simulink model "Non_Holonomical_Cubli"  (R2025b)
settings: Solver=ode15s  StartTime=0  StopTime=13  MaxStep=1e-3  MinStep=1e-8  RelTol=1e-3
values from neighbouring files (symbols this model uses):
  m = 1.219    [physical_parameters.mat]    (also in tuning_parameter_corner.mat; tuning_parameter_edge.mat)
undefined symbols (not defined in the file or in its folder): X, Y, Z
libraries: sm_lib x79, nesl_utility x10, simulink x5, simulink_extras x2
(part 1 of 3)
settings Model: Creator=S Sanjay  LastModifiedBy=S Sanjay
settings SolverCC: InitialStep=1e-3  MaxConsecutiveMinStep=1e4
settings DataIOCC: FinalStateName=Edge_Balance  InitialState=Edge_Balance  SaveOperatingPoint=on
settings SFSimCC: SimTargetLang=C++  SimDLTargetLibrary=mkl-dnn
settings ExplorerConfigSet: InternalSimMechanicsExplorerSettings=|
  | <ExplorerConfiguration>
  | 
  |   <canonicalview>default</canonicalview>
  | 
  |   <TilePanel>
  |     <TileInfo>
  |       <Tiles Columns="1" Count="1" Height="608" Rows="1" Width="1340">
  |         <Row Weight="1"/>
  |         <Column Weight="1"/>
  |         <Tile Height="1" Width="1" X="0" Y="0"/>
  |       </Tiles>
  |     </TileInfo>
  |     <SceneInfo>
  |       <SceneViewer>
  |         <IsThisViewStd>
  |           <IsStandardView>off</IsStandardView>
  |           <StandardViewName>Front</StandardViewName>
  |         </IsThisViewStd>
  |         <BGColor>
  |           <R>1</R>
  |           <G>1</G>
  |           <B>1</B>
  |           <A>1</A>
  |         </BGColor>
  |         <Camera>
  |           <DoPerspective>off</DoPerspective>
  |           <Position>
  |             <X>-0.040054821891673767</X>
  |             <Y>-0.70442291530903711</Y>
  |             <Z>0.071525398260554526</Z>
  |           </Position>
  |           <Center>
  |             <X>-0.040054821891673767</X>
  |             <Y>0.074999999999999997</Y>
  |             <Z>0.071525398260554526</Z>
  |           </Center>
  |           <Up>
  |             <X>0</X>
  |             <Y>0</Y>
  |             <Z>1</Z>
  |           </Up>
  |           <XLim>0.15052058136869881</XLim>
  |           <YLim>0.15052058136869881</YLim>
  |           <ViewLimDist>0.01</ViewLimDist>
  |         </Camera>
  |       </SceneViewer>
  |     </SceneInfo>
  |   </TilePanel>
  | 
  |   <MechEditorPanel>
  |     <GfxPanelCameraMap/>
  |     <Cameras/>
  |     <VideoCreator>
  |       <IncludeTiles>All</IncludeTiles>
  |       <IncludeTime>on</IncludeTime>
  |       <IncludeWorldFrame>off</IncludeWorldFrame>
  |       <PlaybackSpeedRatio>1</PlaybackSpeedRatio>
  |       <FrameRate>30</FrameRate>
  |       <FrameSize>[1280, 720]</FrameSize>
  |       <VideoFormat>MPEG4</VideoFormat>
  |     </VideoCreator>
  |   </MechEditorPanel>
  | 
  |   <PlaybackSettings>
  |     <PlaybackSpeedFactor>1</PlaybackSpeedFactor>
  |   </PlaybackSettings>
  | 
  | </ExplorerConfiguration>

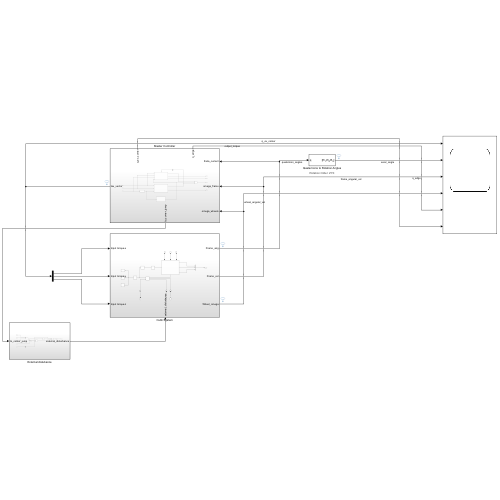
[thumbnail: Simulink's stored preview of the top-level diagram]
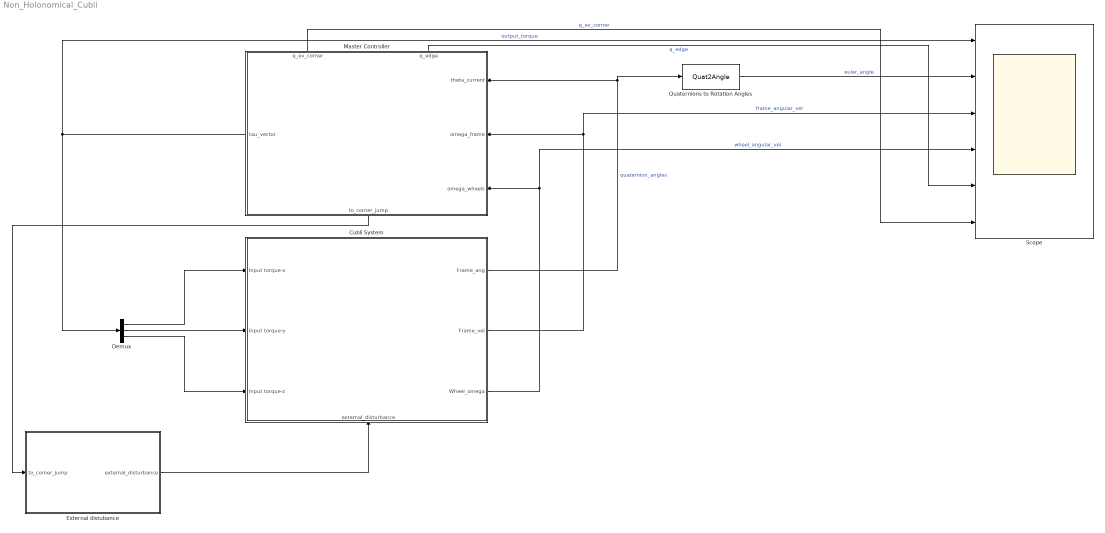
== system Non_Holonomical_Cubli ==
  Cubli System : Subsystem
      settings: PortSchema="{\"entries\":[{\"content\":{\"sides\":[{\"content\":{\"connectorIds\":[\"In1\",\"In2\",\"In3\"]},\"type\":\"ConnectorPlacement.EquallySpacedRectSide\",\"uuid\":\"5f5b9516-a4fd-4785-926f-66a98ec2aae9\"},{\"content\":{\"connectorIds\":[\"Out1\",\"Out2\",\"Out3\"],\"side\":\"RIGHT\"},\"type\":\"ConnectorPlacement.EquallySpacedRectSide\",\"uuid\":\"60d5ee22-f38f-41d5-b6d6-7b831adbf2a8\"},{\"content\":{\"side\":\"TOP\"},\"type\":\"ConnectorPlacement.EquallySpacedRectSide\",\"uuid\":\"7dec9ffc-12fc-4598-886c-49b3d3caf796\"},{\"content\":{\"connectorIds\":[\"In4\"],\"side\":\"BOTTOM\"},\"type\":\"ConnectorPlacement.EquallySpacedRectSide\",\"uuid\":\"6f94ea6b-f13b-4fc8-9dbe-3e3d3e7c7d3e\"}]},\"type\":\"ConnectorPlacement.EquallySpacedConnector\",\"uuid\":\"330043f2-5c26-4a0f-a502-bfb2b6aa9a82\"}],\"packageUris\":[\"http://schema.mathworks.com/mf0/Connector/R2020b\"],\"version\":\"1.0\"}"
  Demux : Demux  Outputs=3
  External distubance : Subsystem
  Master Controller : Subsystem
      settings: PortSchema="{\"entries\":[{\"content\":{\"sides\":[{\"content\":{\"connectorIds\":[\"In1\",\"In2\",\"In3\"]},\"type\":\"ConnectorPlacement.EquallySpacedRectSide\",\"uuid\":\"2cdceb7b-abfe-4398-b06f-eb5d2b1f6282\"},{\"content\":{\"connectorIds\":[\"Out1\"],\"side\":\"RIGHT\"},\"type\":\"ConnectorPlacement.EquallySpacedRectSide\",\"uuid\":\"01c339db-17ac-4119-86eb-536633adac2c\"},{\"content\":{\"connectorIds\":[\"Out3\",\"Out4\"],\"side\":\"TOP\"},\"type\":\"ConnectorPlacement.EquallySpacedRectSide\",\"uuid\":\"b96001bd-d179-4ff4-a950-c514b8b3d76b\"},{\"content\":{\"connectorIds\":[\"Out2\"],\"side\":\"BOTTOM\"},\"type\":\"ConnectorPlacement.EquallySpacedRectSide\",\"uuid\":\"361f408d-891c-47d0-b8eb-9646463b4a1f\"}]},\"type\":\"ConnectorPlacement.EquallySpacedConnector\",\"uuid\":\"bf28b1fe-494a-4ec5-b1bb-391f95a1c354\"}],\"packageUris\":[\"http://schema.mathworks.com/mf0/Connector/R2020b\"],\"version\":\"1.0\"}"
  Quaternions to Rotation Angles : Quat2Angle
      settings: AttributesFormatString=Rotation Order: %<rotationOrder>
  Scope : Scope  NumInputPorts=6
      settings: ActiveDisplayYMinimum=-12.75  ActiveDisplayYMaximum=24.75
  wires:
  Cubli System/1(Frame_ang) -> Quaternions to Rotation Angles/1, Master Controller/1(theta_current)  "quaternion_angles"
  Cubli System/2(Frame_vel) -> Scope/3, Master Controller/2(omega_frame)  "frame_angular_vel"
  Cubli System/3(Wheel_omega) -> Scope/4, Master Controller/3(omega_wheels)  "wheel_angular_vel"
  Master Controller/1(tau_vector) -> Scope/1, Demux/1  "output_torque"
  Demux/1 -> Cubli System/1(Input torque-x)
  Demux/2 -> Cubli System/2(Input torque-y)
  Demux/3 -> Cubli System/3(Input torque-z)
  Master Controller/3(q_edge) -> Scope/5  "q_edge"
  Master Controller/4(q_ev_corner) -> Scope/6  "q_ev_corner"
  Quaternions to Rotation Angles/1 -> Scope/2  "euler_angle"
  Master Controller/2(to_corner_jump) -> External distubance/1(to_corner_jump)
  External distubance/1(external_disturbance) -> Cubli System/4(external_disturbance)

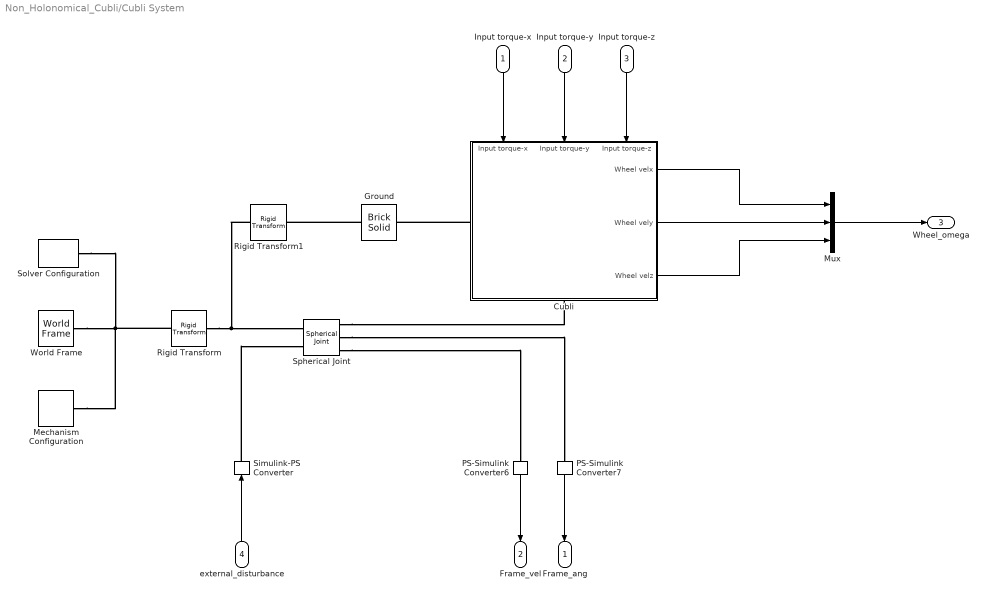
== system Non_Holonomical_Cubli/Cubli System ==
  Input torque-x : Inport
  Input torque-y : Inport  Port=2
  Input torque-z : Inport  Port=3
  external_disturbance : Inport  Port=4
  Cubli : Subsystem
      settings: PortSchema="{\"entries\":[{\"content\":{\"sides\":[{\"content\":{\"connectorIds\":[\"LConn1\"]},\"type\":\"ConnectorPlacement.EquallySpacedRectSide\",\"uuid\":\"6adf7ee2-c4b8-4796-ad09-ce5711974701\"},{\"content\":{\"connectorIds\":[\"Out1\",\"Out2\",\"Out3\"],\"side\":\"RIGHT\"},\"type\":\"ConnectorPlacement.EquallySpacedRectSide\",\"uuid\":\"91dc68f1-4c76-44e8-ad07-f96271bd7b17\"},{\"content\":{\"connectorIds\":[\"In1\",\"In2\",\"In3\"],\"side\":\"TOP\"},\"type\":\"ConnectorPlacement.EquallySpacedRectSide\",\"uuid\":\"30232ce5-1395-4c39-8bb0-085fb3773f51\"},{\"content\":{\"connectorIds\":[\"RConn1\"],\"side\":\"BOTTOM\"},\"type\":\"ConnectorPlacement.EquallySpacedRectSide\",\"uuid\":\"0f945396-4cf4-432c-84ba-6526ad05d30a\"}]},\"type\":\"ConnectorPlacement.EquallySpacedConnector\",\"uuid\":\"10f6f1ea-d2be-46df-87d0-79c43156557a\"}],\"packageUris\":[\"http://schema.mathworks.com/mf0/Connector/R2020b\"],\"version\":\"1.0\"}"
  Ground : sm_lib/Body Elements/Brick Solid  BrickDimensions=[1 1 0.02]  BrickDimensionsUnits=m  ExportEntireGeometry=on  InertiaType=CalculateFromGeometry  BasedOnType=Density  Density=1000  DensityUnits=kg/m^3  Mass=1  MassUnits=kg  CenterOfMass=[0 0 0]  CenterOfMassUnits=m  MomentsOfInertia=[1 1 1]  MomentsOfInertiaUnits=kg*m^2  ProductsOfInertia=[0 0 0]  ProductsOfInertiaUnits=kg*m^2  GraphicType=FromGeometry  MarkerShape=Sphere  MarkerSize=10  GraphicVisPropType=SimpleVisualProperties  GraphicDiffuseColor=[0.5 0.5 0.5]  GraphicOpacity=1  GraphicSpecularColor=[0.5 0.5 0.5 1.0]  GraphicAmbientColor=[0.15 0.15 0.15 1.0]  GraphicEmissiveColor=[0.0 0.0 0.0 1.0]  GraphicShininess=75  DoExposeReferenceFrame=on  SerializedFrames=<Frames/>
  Mechanism Configuration : sm_lib/Utilities/Mechanism Configuration  UniformGravity=Constant  GravityVector=[0 0 -9.80665]  GravityVectorUnits=m/s^2  LinearizationDelta=0.001  JointModeTransitionNonlinearIterations=2
  Mux : Mux  Inputs=3
  PS-Simulink Converter6 : nesl_utility/PS-Simulink Converter  PhysicalDomain=network_engine_domain  SubClassName=ps_output  LeftPortType=input  RightPortType=output  PseudoPeriodic=off  Frequencies=[]  VectorFormat=inherit  Unit=inherit  AffineConversion=off
  PS-Simulink Converter7 : nesl_utility/PS-Simulink Converter  PhysicalDomain=network_engine_domain  SubClassName=ps_output  LeftPortType=input  RightPortType=output  PseudoPeriodic=off  Frequencies=[]  VectorFormat=inherit  Unit=inherit  AffineConversion=off
  Rigid Transform : sm_lib/Frames and Transforms/Rigid Transform  RotationMethod=None  FollAlignAxisA=+X  BaseAlignAxisA=+Y  FollAlignAxisB=+Y  BaseAlignAxisB=+Z  RotationStandardAxis=+X  RotationAngle=90  RotationAngleUnits=deg  RotationArbitraryAxis=[0 0 1]  RotationSequenceAxes=FollowerAxes  RotationSequence=XYX  RotationSequenceAngles=[90 180 0]  RotationSequenceAnglesUnits=deg  RotationMatrix=[1 0 0;0 1 0;0 0 1]  Quaternion=[1 0 0 0]  TranslationMethod=None  TranslationCartesianOffset=[0 0 0]  TranslationCartesianOffsetUnits=m  TranslationStandardAxis=+Z  TranslationStandardOffset=0  TranslationStandardOffsetUnits=m  TranslationROffset=0  TranslationROffsetUnits=m  TranslationThetaOffset=0  TranslationThetaOffsetUnits=deg  TranslationZOffset=0  TranslationZOffsetUnits=m
  Rigid Transform1 : sm_lib/Frames and Transforms/Rigid Transform  RotationMethod=None  FollAlignAxisA=+X  BaseAlignAxisA=+Y  FollAlignAxisB=+Y  BaseAlignAxisB=+Z  RotationStandardAxis=+X  RotationAngle=90  RotationAngleUnits=deg  RotationArbitraryAxis=[0 0 1]  RotationSequenceAxes=FollowerAxes  RotationSequence=XYX  RotationSequenceAngles=[90 180 0]  RotationSequenceAnglesUnits=deg  RotationMatrix=[1 0 0;0 1 0;0 0 1]  Quaternion=[1 0 0 0]  TranslationMethod=StandardAxis  TranslationCartesianOffset=[0 0 0]  TranslationCartesianOffsetUnits=m  TranslationStandardAxis=+Z  TranslationStandardOffset=-0.01  TranslationStandardOffsetUnits=m  TranslationROffset=0  TranslationROffsetUnits=m  TranslationThetaOffset=0  TranslationThetaOffsetUnits=deg  TranslationZOffset=0  TranslationZOffsetUnits=m
  Simulink-PS Converter : nesl_utility/Simulink-PS Converter  PhysicalDomain=network_engine_domain  SubClassName=ps_input  LeftPortType=input  RightPortType=output  PseudoPeriodic=off  Frequencies=[]  NoiseDistribution=none  NoiseParameters=[]  Unit=1  AffineConversion=off  FilteringAndDerivatives=provide  SimscapeFilterOrder=1  InputFilterTimeConstant=0.001  UdotUserProvided=0
  Solver Configuration : nesl_utility/Solver Configuration  PhysicalDomain=network_engine_domain  SubClassName=solver  LeftPortType=input  RightPortType=generic  Tones=[]  Harmonics=[]  SimulateNoise=off  Profile=off  UseLocalSampling=off  EnableSwitchedLinearOptims=on  FrequencyDomain=off  UseCCode=off  RelTol=0.001  AbsTol=0.001  MinStep=1e-09  ToWorkspace=off  RevertToSquareIcSolve=off  NumHomotopyIterations=100  PhasorMode=off  PhasorModeNumHarmonics=1  ConsistencySolver=NEWTON_XTOL_AFTER_FTOL  IndexReductionMethod=DerivativeReplacement  DoDC=off  ResidualTolerance=1e-09  ConsistencyTolSource=GLOBAL  ConsistencyAbsTol=0.001  ConsistencyRelTol=0.001  ConsistencyTolFactor=0.001  UseLocalSolver=off  LocalSolverChoice=NE_BACKWARD_EULER_ADVANCER  ResolveIndetEquations=on  FunctionEvalNumThread=1  LocalSolverSampleTime=0.001  DoFixedCost=off  MaxNonlinIter=3  MaxModeIter=2  ComputeImpulses=off  ImpulseIterations=2  LinearAlgebra=auto  LinearAlgebraNumThread=0  EquationFormulation=NE_TIME_EF  DelaysMemoryBudget=1024  AutomaticFiltering=on  FilteringTimeConstant=0.001  PartitionStorageMethod=AS_NEEDED  PartitionMemoryBudget=1024  PartitionMethod=ROBUST  MultibodyUseLocalSolver=off  MultibodyLocalSolverChoice=ODE1  MultibodyLocalSolverSampleTime=0.001
  Spherical Joint : sm_lib/Joints/Spherical Joint  JointMode=Normal  CompositeWrenchDir=FollowerOnBase  CompositeWrenchFrame=BaseFrame  SenseConstraintForce=off  SenseConstraintTorque=off  SenseTotalForce=off  SenseTotalTorque=off  PositionTargetSpecify=on  PositionTargetPriority=High  PositionTargetRotationMethod=RotationSequence  PositionTargetFollAlignAxisA=+X  PositionTargetBaseAlignAxisA=+Y  PositionTargetFollAlignAxisB=+Y  PositionTargetBaseAlignAxisB=+Z  PositionTargetRotationStandardAxis=+Z  PositionTargetRotationAngle=0  PositionTargetRotationAngleUnits=deg  PositionTargetRotationArbitraryAxis=[0 0 1]  PositionTargetRotationSequenceAxes=BaseAxes  PositionTargetRotationSequence=XYX  PositionTargetRotationSequenceAngles=[0 -05 0]  PositionTargetRotationSequenceAnglesUnits=deg  PositionTargetRotationMatrix=[1 0 0;0 1 0;0 0 1]  PositionTargetQuaternion=[1 0 0 0]  VelocityTargetSpecify=off  VelocityTargetPriority=High  VelocityTargetValue=[7.592 0.1228 0.0118]  VelocityTargetValueUnits=rad/s  VelocityTargetInFollowerFrame=off  EqPosRotationMethod=None  EqPosFollAlignAxisA=+X  EqPosBaseAlignAxisA=+Y  EqPosFollAlignAxisB=+Y  EqPosBaseAlignAxisB=+Z  EqPosRotationStandardAxis=+Z  EqPosRotationAngle=0  EqPosRotationAngleUnits=deg  EqPosRotationArbitraryAxis=[0 0 1]  EqPosRotationSequenceAxes=FollowerAxes  EqPosRotationSequence=XYX  EqPosRotationSequenceAngles=[0 0 0]  EqPosRotationSequenceAnglesUnits=deg  EqPosRotationMatrix=[1 0 0;0 1 0;0 0 1]  EqPosQuaternion=[1 0 0 0]  SpringStiffness=0  SpringStiffnessUnits=N*m/deg  DampingCoefficient=0.01  DampingCoefficientUnits=N*m/(deg/s)  LowerLimitSpecify=off  LowerLimitBound=15  LowerLimitBoundUnits=deg  LowerLimitStiffness=1e4  LowerLimitStiffnessUnits=N*m/deg  LowerLimitDamping=10  LowerLimitDampingUnits=N*m/(deg/s)  LowerLimitTransitionRegionWidth=0.1  LowerLimitTransitionRegionWidthUnits=deg  UpperLimitSpecify=off  UpperLimitBound=45  UpperLimitBoundUnits=deg  UpperLimitStiffness=1e4  UpperLimitStiffnessUnits=N*m/deg  UpperLimitDamping=10  UpperLimitDampingUnits=N*m/(deg/s)  UpperLimitTransitionRegionWidth=0.1  UpperLimitTransitionRegionWidthUnits=deg  TorqueActuationMode=InputTorque  ActuateTorqueX=off  ActuateTorqueY=off  ActuateTorqueZ=off  ActuateTorque=on  ActuationFrame=BaseFrame  SensePosition=on  SenseVelocityX=off  SenseVelocityY=off  SenseVelocityZ=off  SenseVelocity=on  SenseAccelerationX=off  SenseAccelerationY=off  SenseAccelerationZ=off  SenseAcceleration=off  SenseLowerLimitTorqueMag=off  SenseUpperLimitTorqueMag=off  SensingFrame=BaseFrame
  World Frame : sm_lib/Frames and Transforms/World Frame
  Frame_ang : Outport
  Frame_vel : Outport  Port=2
  Wheel_omega : Outport  Port=3
  wires:
  Input torque-z/1 -> Cubli/3(Input torque-z)
  Input torque-y/1 -> Cubli/2(Input torque-y)
  Input torque-x/1 -> Cubli/1(Input torque-x)
  Cubli/2(Wheel vely) -> Mux/2
  Cubli/1(Wheel velx) -> Mux/1
  Cubli/3(Wheel velz) -> Mux/3
  Mux/1 -> Wheel_omega/1
  PS-Simulink Converter6/1 -> Frame_vel/1
  PS-Simulink Converter7/1 -> Frame_ang/1
  external_disturbance/1 -> Simulink-PS Converter/1
  connections:
  World Frame/RConn1 -- Rigid Transform/LConn1 -- Solver Configuration/RConn1 -- Mechanism Configuration/RConn1
  Spherical Joint/RConn1 -- Cubli/RConn1
  Rigid Transform/RConn1 -- Rigid Transform1/LConn1 -- Spherical Joint/LConn1
  Spherical Joint/RConn3 -- PS-Simulink Converter6/LConn1
  Spherical Joint/RConn2 -- PS-Simulink Converter7/LConn1
  Ground/RConn1 -- Rigid Transform1/RConn1
  Cubli/LConn1 -- Ground/LConn1
  Simulink-PS Converter/RConn1 -- Spherical Joint/LConn2

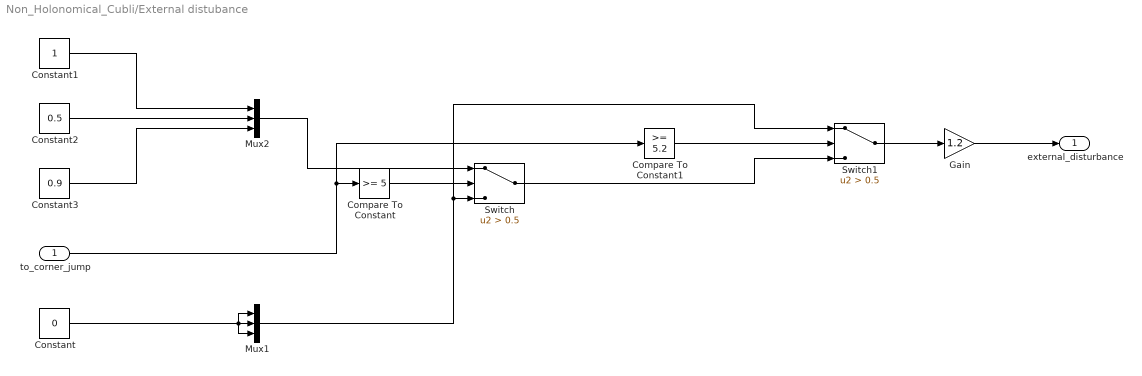
== system Non_Holonomical_Cubli/External distubance ==
  to_corner_jump : Inport
  Compare To Constant : simulink/Logic and Bit Operations/Compare To Constant  relop=>=  const=5  OutDataTypeStr=boolean
  Compare To Constant1 : simulink/Logic and Bit Operations/Compare To Constant  relop=>=  const=5.2  OutDataTypeStr=boolean
  Constant : Constant  Value=0
  Constant1 : Constant
  Constant2 : Constant  Value=0.5
  Constant3 : Constant  Value=0.9
  Gain : Gain  Gain=1.2
  Mux1 : Mux  Inputs=3
  Mux2 : Mux  Inputs=3
  Switch : Switch  Criteria=u2 > Threshold  Threshold=0.5  SaturateOnIntegerOverflow=off  InputSameDT=off
  Switch1 : Switch  Criteria=u2 > Threshold  Threshold=0.5  SaturateOnIntegerOverflow=off  InputSameDT=off
  external_disturbance : Outport
  wires:
  Compare To Constant/1 -> Switch/2
  to_corner_jump/1 -> Compare To Constant/1, Compare To Constant1/1
  Switch/1 -> Switch1/3
  Constant1/1 -> Mux2/1
  Constant/1 -> Mux1/3, Mux1/1, Mux1/2
  Mux1/1 -> Switch1/1, Switch/3
  Compare To Constant1/1 -> Switch1/2
  Constant2/1 -> Mux2/2
  Constant3/1 -> Mux2/3
  Switch1/1 -> Gain/1
  Mux2/1 -> Switch/1
  Gain/1 -> external_disturbance/1

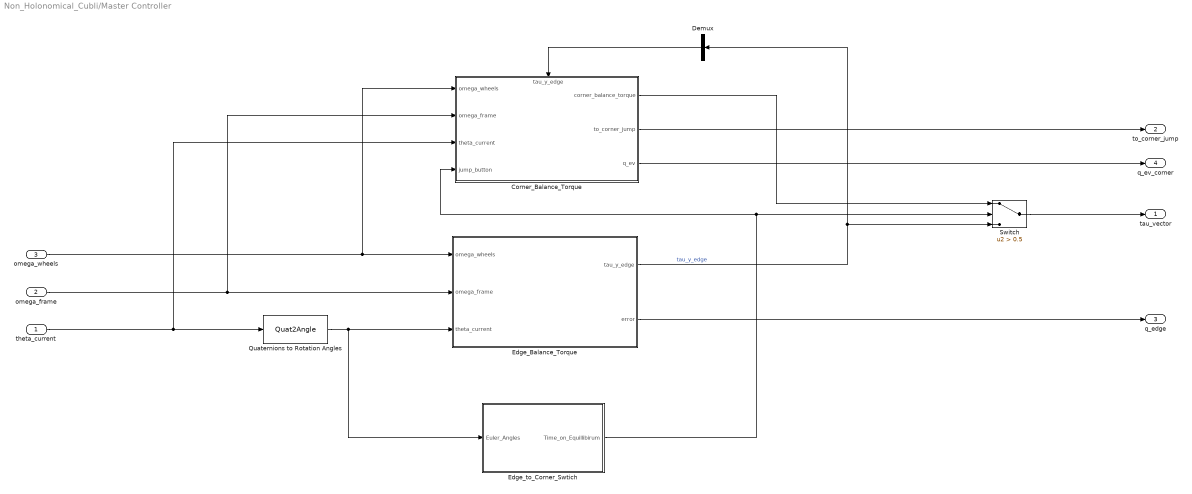
== system Non_Holonomical_Cubli/Master Controller ==
  theta_current : Inport
  omega_frame : Inport  Port=2
  omega_wheels : Inport  Port=3
  Corner_Balance_Torque : Subsystem
      settings: PortSchema="{\"entries\":[{\"content\":{\"sides\":[{\"content\":{\"connectorIds\":[\"In1\",\"In2\",\"In3\",\"In4\"]},\"type\":\"ConnectorPlacement.EquallySpacedRectSide\",\"uuid\":\"1f7b0852-8b9a-4eba-b230-002f04ce1124\"},{\"content\":{\"connectorIds\":[\"Out1\",\"Out2\",\"Out3\"],\"side\":\"RIGHT\"},\"type\":\"ConnectorPlacement.EquallySpacedRectSide\",\"uuid\":\"21919282-dafc-4587-878f-e5107e503542\"},{\"content\":{\"connectorIds\":[\"In5\"],\"side\":\"TOP\"},\"type\":\"ConnectorPlacement.EquallySpacedRectSide\",\"uuid\":\"4f05e2a3-4b7f-447f-b0fe-b8f447574882\"}]},\"type\":\"ConnectorPlacement.EquallySpacedConnector\",\"uuid\":\"49aab782-7a49-4f61-ae94-efa1138c681a\"}],\"packageUris\":[\"http://schema.mathworks.com/mf0/Connector/R2020b\"],\"version\":\"1.0\"}"
  Demux : Demux  Outputs=3
  Edge_Balance_Torque : Subsystem
  Edge_to_Corner_Swtich : Subsystem
  Quaternions to Rotation Angles : Quat2Angle
      settings: AttributesFormatString=Rotation Order: %<rotationOrder>
  Switch : Switch  Criteria=u2 > Threshold  Threshold=0.5  SaturateOnIntegerOverflow=off  InputSameDT=off
  tau_vector : Outport
  to_corner_jump : Outport  Port=2
  q_edge : Outport  Port=3
  q_ev_corner : Outport  Port=4
  wires:
  omega_frame/1 -> Corner_Balance_Torque/2(omega_frame), Edge_Balance_Torque/2(omega_frame)
  omega_wheels/1 -> Corner_Balance_Torque/1(omega_wheels), Edge_Balance_Torque/1(omega_wheels)
  Edge_Balance_Torque/2(error) -> q_edge/1
  theta_current/1 -> Quaternions to Rotation Angles/1, Corner_Balance_Torque/3(theta_current)
  Quaternions to Rotation Angles/1 -> Edge_to_Corner_Swtich/1(Euler_Angles), Edge_Balance_Torque/3(theta_current)
  Corner_Balance_Torque/1(corner_balance_torque) -> Switch/1
  Switch/1 -> tau_vector/1
  Edge_to_Corner_Swtich/1(Time_on_Equillibirum) -> Switch/2, Corner_Balance_Torque/4(jump_button)
  Edge_Balance_Torque/1(tau_y_edge) -> Demux/1, Switch/3  "tau_y_edge"
  Demux/2 -> Corner_Balance_Torque/5(tau_y_edge)
  Corner_Balance_Torque/2(to_corner_jump) -> to_corner_jump/1
  Corner_Balance_Torque/3(q_ev) -> q_ev_corner/1

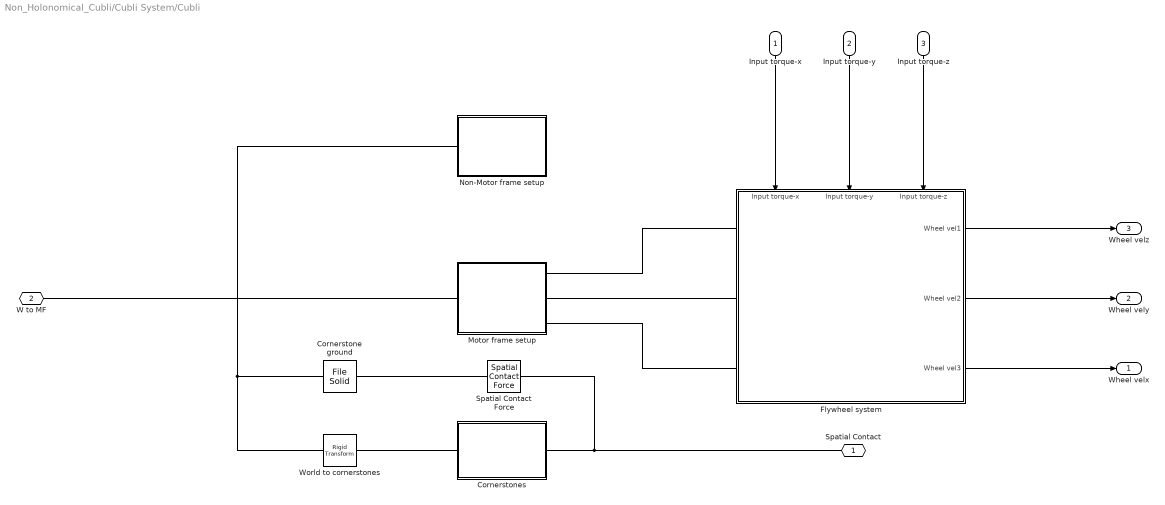
== system Non_Holonomical_Cubli/Cubli System/Cubli ==
  Input torque-x : Inport
  Input torque-y : Inport  Port=2
  Input torque-z : Inport  Port=3
  Cornerstone ground : sm_lib/Body Elements/File Solid  ExtGeomFileName=D:\Mechatronics\Non-Holonomical Cubli\GitHub Referance\balancing-cube-main\mechanical\models\cornerstone-b.step  UnitType=FromFile  ExtGeomFileUnits=m  StepReaderType=HEX  ExportConvexHullGeometry=on  InertiaType=Custom  BasedOnType=DensityFromFile  Density=1000  DensityUnits=kg/m^3  Mass=15.195  MassUnits=g  CenterOfMass=[7.102 7.102 7.102]  CenterOfMassUnits=mm  MomentsOfInertia=[4.91955e-7 4.91955e-7 4.91955e-7]  MomentsOfInertiaUnits=kg*m^2  ProductsOfInertia=[2.9611e-8 2.9611e-8 2.9611e-8]  ProductsOfInertiaUnits=kg*m^2  GraphicType=FromGeometry  MarkerShape=Sphere  MarkerSize=10  GraphicVisPropType=SimpleVisualProperties  GraphicDiffuseColor=[0 0.7137 0.02353]  GraphicOpacity=1  GraphicSpecularColor=[0.5 0.5 0.5 1.0]  GraphicAmbientColor=[0.15 0.15 0.15 1.0]  GraphicEmissiveColor=[0.0 0.0 0.0 1.0]  GraphicShininess=75  DoExposeReferenceFrame=on  SerializedFrames=<Frames/>
  Cornerstones : Subsystem
  Flywheel system : Subsystem
      settings: PortSchema="{\"entries\":[{\"content\":{\"sides\":[{\"content\":{\"connectorIds\":[\"LConn1\",\"LConn2\",\"LConn3\"]},\"type\":\"ConnectorPlacement.EquallySpacedRectSide\",\"uuid\":\"bd01766a-4f70-4c8a-b3da-7a2c61393a0a\"},{\"content\":{\"connectorIds\":[\"Out1\",\"Out2\",\"Out3\"],\"side\":\"RIGHT\"},\"type\":\"ConnectorPlacement.EquallySpacedRectSide\",\"uuid\":\"6c934dc6-4dcb-4252-8a96-3382836f91aa\"},{\"content\":{\"connectorIds\":[\"In1\",\"In2\",\"In3\"],\"side\":\"TOP\"},\"type\":\"ConnectorPlacement.EquallySpacedRectSide\",\"uuid\":\"3baafda2-b803-466a-93fa-ff8a48a98b9a\"}]},\"type\":\"ConnectorPlacement.EquallySpacedConnector\",\"uuid\":\"eb6514d5-6f26-4cfd-b495-999f94607100\"}],\"packageUris\":[\"http://schema.mathworks.com/mf0/Connector/R2020b\"],\"version\":\"1.0\"}"
  Motor frame setup : Subsystem
  Non-Motor frame setup : Subsystem
  Spatial Contact Force : sm_lib/Forces and Torques/Spatial Contact Force  SenseSeparationDistance=off  NormalForceType=SmoothSpringDamper  NormalStiffness=1e6  NormalStiffnessUnits=N/m  NormalDamping=1e3  NormalDampingUnits=N/(m/s)  NormalTransitionRegionWidth=1e-4  NormalTransitionRegionWidthUnits=m  FrictionType=SmoothStickSlip  CoefficientOfStaticFriction=0.5  CoefficientOfDynamicFriction=0.3  FrictionalCriticalVelocity=1e-3  FrictionalCriticalVelocityUnits=m/s  SenseContactSignal=off  SensePenetrationDepth=off  SenseNormalVelocity=off  SenseTangentialVelocity=off  SensingForceTorqueDirection=BaseOnFollower  SensingForceTorqueResolutionFrame=ContactFrame  SenseNormalForce=off  SenseNormalForceMagnitude=off  SenseNormalTorque=off  SenseFrictionalForce=off  SenseFrictionalForceMagnitude=off  SenseFrictionalTorque=off  SenseTotalForce=off  SenseTotalTorque=off  SenseContactBaseRotation=off  SenseContactBaseTranslation=off  SenseContactFollowerRotation=off  SenseContactFollowerTranslation=off  ZeroCrossDetectContactStartAndEnd=off
  World to cornerstones : sm_lib/Frames and Transforms/Rigid Transform  RotationMethod=StandardAxis  FollAlignAxisA=+X  BaseAlignAxisA=+Y  FollAlignAxisB=+Y  BaseAlignAxisB=+Z  RotationStandardAxis=+Z  RotationAngle=180  RotationAngleUnits=deg  RotationArbitraryAxis=[0 0 1]  RotationSequenceAxes=FollowerAxes  RotationSequence=XZY  RotationSequenceAngles=[0 0 0]  RotationSequenceAnglesUnits=deg  RotationMatrix=[1 0 0;0 1 0;0 0 1]  Quaternion=[1 0 0 0]  TranslationMethod=Cartesian  TranslationCartesianOffset=[75 75 0]  TranslationCartesianOffsetUnits=mm  TranslationStandardAxis=+Z  TranslationStandardOffset=0  TranslationStandardOffsetUnits=m  TranslationROffset=0  TranslationROffsetUnits=m  TranslationThetaOffset=0  TranslationThetaOffsetUnits=deg  TranslationZOffset=0  TranslationZOffsetUnits=m
  Spatial Contact : PMIOPort  Side=Left
  W to MF : PMIOPort  Port=2  Side=Right
  Wheel velx : Outport
  Wheel vely : Outport  Port=2
  Wheel velz : Outport  Port=3
  wires:
  Flywheel system/1(Wheel vel1) -> Wheel velz/1
  Input torque-z/1 -> Flywheel system/3(Input torque-z)
  Flywheel system/3(Wheel vel3) -> Wheel velx/1
  Flywheel system/2(Wheel vel2) -> Wheel vely/1
  Input torque-x/1 -> Flywheel system/1(Input torque-x)
  Input torque-y/1 -> Flywheel system/2(Input torque-y)
  connections:
  World to cornerstones/LConn1 -- Non-Motor frame setup/LConn1 -- W to MF/RConn1 -- Motor frame setup/LConn1 -- Cornerstone ground/RConn1
  Cornerstones/LConn1 -- World to cornerstones/RConn1
  Flywheel system/LConn2 -- Motor frame setup/RConn2
  Flywheel system/LConn1 -- Motor frame setup/RConn1
  Flywheel system/LConn3 -- Motor frame setup/RConn3
  Spatial Contact/RConn1 -- Spatial Contact Force/LConn1 -- Cornerstones/RConn1
  Spatial Contact Force/RConn1 -- Cornerstone ground/LConn1

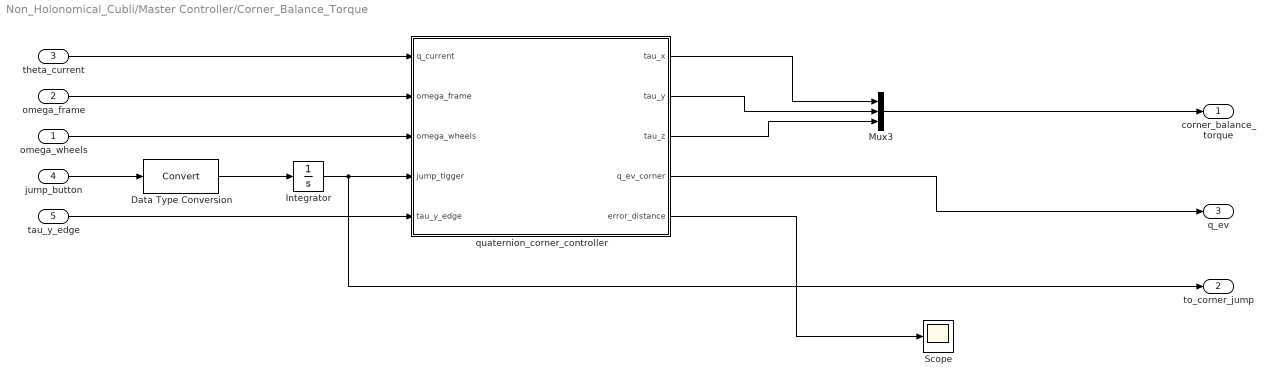
== system Non_Holonomical_Cubli/Master Controller/Corner_Balance_Torque ==
  omega_wheels : Inport
  omega_frame : Inport  Port=2
  theta_current : Inport  Port=3
  jump_button : Inport  Port=4
  tau_y_edge : Inport  Port=5
  Data Type Conversion : DataTypeConversion  SaturateOnIntegerOverflow=off  RndMeth=Floor
  Integrator : Integrator
  Mux3 : Mux  Inputs=3
  Scope : Scope
      settings: ActiveDisplayYMinimum=-0.059292060386496544  ActiveDisplayYMaximum=0.53363013219783351
  quaternion_corner_controller : MATLAB Function  TreatAsAtomicUnit=on
  corner_balance_torque : Outport
  to_corner_jump : Outport  Port=2
  q_ev : Outport  Port=3
  wires:
  omega_frame/1 -> quaternion_corner_controller/2(omega_frame)
  omega_wheels/1 -> quaternion_corner_controller/3(omega_wheels)
  quaternion_corner_controller/2(tau_y) -> Mux3/2
  quaternion_corner_controller/1(tau_x) -> Mux3/1
  quaternion_corner_controller/3(tau_z) -> Mux3/3
  Mux3/1 -> corner_balance_torque/1
  tau_y_edge/1 -> quaternion_corner_controller/5(tau_y_edge)
  jump_button/1 -> Data Type Conversion/1
  Integrator/1 -> to_corner_jump/1, quaternion_corner_controller/4(jump_tigger)
  Data Type Conversion/1 -> Integrator/1
  theta_current/1 -> quaternion_corner_controller/1(q_current)
  quaternion_corner_controller/4(q_ev_corner) -> q_ev/1
  quaternion_corner_controller/5(error_distance) -> Scope/1

== system Non_Holonomical_Cubli/Master Controller/Edge_Balance_Torque ==
  omega_wheels : Inport
  omega_frame : Inport  Port=2
  theta_current : Inport  Port=3
  Edge_SMC : MATLAB Function  TreatAsAtomicUnit=on
  Mux : Mux  Inputs=3
  jump_switch : Subsystem
  tau_y_edge : Outport
  error : Outport  Port=2
  wires:
  Edge_SMC/4(error_distance) -> error/1
  omega_frame/1 -> Edge_SMC/2(omega_frame)
  omega_wheels/1 -> Edge_SMC/3(omega_wheels)
  theta_current/1 -> jump_switch/1(theta_angle), Edge_SMC/1(theta_current)
  Edge_SMC/2(tau_y) -> Mux/2
  Edge_SMC/1(tau_x) -> Mux/1
  Edge_SMC/3(tau_z) -> Mux/3
  jump_switch/1(timmer) -> Edge_SMC/4(jump_trigger)
  Mux/1 -> tau_y_edge/1

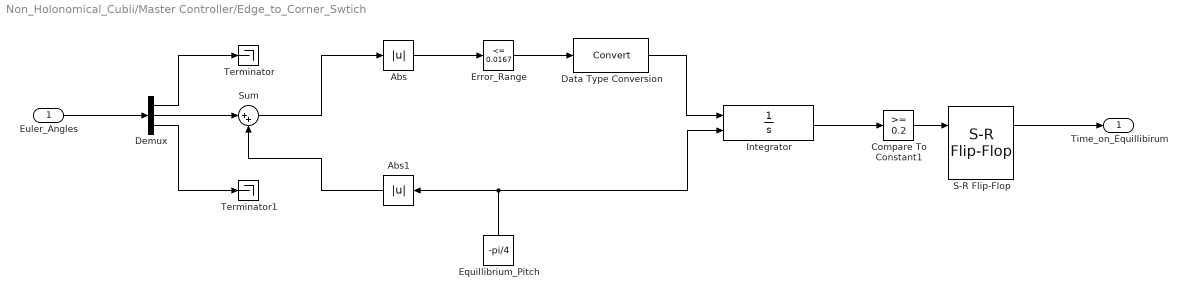
== system Non_Holonomical_Cubli/Master Controller/Edge_to_Corner_Swtich ==
  Euler_Angles : Inport
  Abs : Abs  SaturateOnIntegerOverflow=off
  Abs1 : Abs  SaturateOnIntegerOverflow=off
  Compare To Constant1 : simulink/Logic and Bit Operations/Compare To Constant  relop=>=  const=0.2  OutDataTypeStr=boolean
  Data Type Conversion : DataTypeConversion  SaturateOnIntegerOverflow=off  RndMeth=Floor
  Demux : Demux  Outputs=3
  Equillibrium_Pitch : Constant  Value=-pi/4
  Error_Range : simulink/Logic and Bit Operations/Compare To Constant  relop=<=  const=0.0167  OutDataTypeStr=boolean
  Integrator : Integrator  ExternalReset=falling
  S-R Flip-Flop : simulink_extras/Flip Flops/S-R Flip-Flop  initial_condition=0
  Sum : Sum  Inputs=|++
  Terminator : Terminator
  Terminator1 : Terminator
  Time_on_Equillibirum : Outport
  wires:
  Compare To Constant1/1 -> S-R Flip-Flop/1
  Equillibrium_Pitch/1 -> Integrator/2, Abs1/1
  Abs/1 -> Error_Range/1
  Abs1/1 -> Sum/2
  Data Type Conversion/1 -> Integrator/1
  Error_Range/1 -> Data Type Conversion/1
  Demux/2 -> Sum/1
  Integrator/1 -> Compare To Constant1/1
  Sum/1 -> Abs/1
  Demux/3 -> Terminator1/1
  Demux/1 -> Terminator/1
  S-R Flip-Flop/1 -> Time_on_Equillibirum/1
  Euler_Angles/1 -> Demux/1

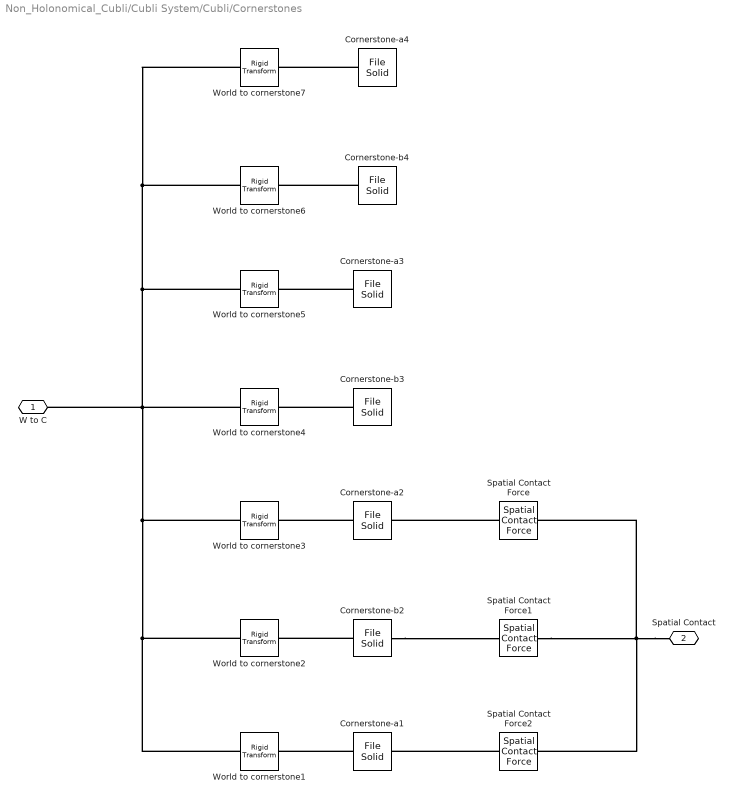
== system Non_Holonomical_Cubli/Cubli System/Cubli/Cornerstones ==
  Cornerstone-a1 : sm_lib/Body Elements/File Solid  ExtGeomFileName=D:\Mechatronics\Non-Holonomical Cubli\GitHub Referance\balancing-cube-main\mechanical\models\cornerstone-a.step  UnitType=FromFile  ExtGeomFileUnits=m  StepReaderType=HEX  ExportConvexHullGeometry=on  InertiaType=Custom  BasedOnType=DensityFromFile  Density=1000  DensityUnits=kg/m^3  Mass=15.195  MassUnits=g  CenterOfMass=[7.102 7.102 7.102]  CenterOfMassUnits=mm  MomentsOfInertia=[4.91955e-7 4.91955e-7 4.91955e-7]  MomentsOfInertiaUnits=kg*m^2  ProductsOfInertia=[2.9611e-8 2.9611e-8 2.9611e-8]  ProductsOfInertiaUnits=kg*m^2  GraphicType=FromGeometry  MarkerShape=Sphere  MarkerSize=10  GraphicVisPropType=SimpleVisualProperties  GraphicDiffuseColor=[0 0.7137 0.02353]  GraphicOpacity=1  GraphicSpecularColor=[0.5 0.5 0.5 1.0]  GraphicAmbientColor=[0.15 0.15 0.15 1.0]  GraphicEmissiveColor=[0.0 0.0 0.0 1.0]  GraphicShininess=75  DoExposeReferenceFrame=on  SerializedFrames=<Frames/>
  Cornerstone-a2 : sm_lib/Body Elements/File Solid  ExtGeomFileName=D:\Mechatronics\Non-Holonomical Cubli\GitHub Referance\balancing-cube-main\mechanical\models\cornerstone-a.step  UnitType=FromFile  ExtGeomFileUnits=m  StepReaderType=HEX  ExportConvexHullGeometry=on  InertiaType=Custom  BasedOnType=DensityFromFile  Density=1000  DensityUnits=kg/m^3  Mass=15.195  MassUnits=g  CenterOfMass=[7.102 7.102 7.102]  CenterOfMassUnits=mm  MomentsOfInertia=[4.91955e-7 4.91955e-7 4.91955e-7]  MomentsOfInertiaUnits=kg*m^2  ProductsOfInertia=[2.9611e-8 2.9611e-8 2.9611e-8]  ProductsOfInertiaUnits=kg*m^2  GraphicType=FromGeometry  MarkerShape=Sphere  MarkerSize=10  GraphicVisPropType=SimpleVisualProperties  GraphicDiffuseColor=[0 0.7137 0.02353]  GraphicOpacity=1  GraphicSpecularColor=[0.5 0.5 0.5 1.0]  GraphicAmbientColor=[0.15 0.15 0.15 1.0]  GraphicEmissiveColor=[0.0 0.0 0.0 1.0]  GraphicShininess=75  DoExposeReferenceFrame=on  SerializedFrames=<Frames/>
  Cornerstone-a3 : sm_lib/Body Elements/File Solid  ExtGeomFileName=D:\Mechatronics\Non-Holonomical Cubli\GitHub Referance\balancing-cube-main\mechanical\models\cornerstone-a.step  UnitType=FromFile  ExtGeomFileUnits=m  StepReaderType=HEX  ExportConvexHullGeometry=off  InertiaType=Custom  BasedOnType=DensityFromFile  Density=1000  DensityUnits=kg/m^3  Mass=15.195  MassUnits=g  CenterOfMass=[7.102 7.102 7.102]  CenterOfMassUnits=mm  MomentsOfInertia=[4.91955e-7 4.91955e-7 4.91955e-7]  MomentsOfInertiaUnits=kg*m^2  ProductsOfInertia=[2.9611e-8 2.9611e-8 2.9611e-8]  ProductsOfInertiaUnits=kg*m^2  GraphicType=FromGeometry  MarkerShape=Sphere  MarkerSize=10  GraphicVisPropType=SimpleVisualProperties  GraphicDiffuseColor=[0 0.7137 0.02353]  GraphicOpacity=1  GraphicSpecularColor=[0.5 0.5 0.5 1.0]  GraphicAmbientColor=[0.15 0.15 0.15 1.0]  GraphicEmissiveColor=[0.0 0.0 0.0 1.0]  GraphicShininess=75  DoExposeReferenceFrame=on  SerializedFrames=<Frames/>
  Cornerstone-a4 : sm_lib/Body Elements/File Solid  ExtGeomFileName=D:\Mechatronics\Non-Holonomical Cubli\GitHub Referance\balancing-cube-main\mechanical\models\cornerstone-a.step  UnitType=FromFile  ExtGeomFileUnits=m  StepReaderType=HEX  ExportConvexHullGeometry=off  InertiaType=Custom  BasedOnType=DensityFromFile  Density=1000  DensityUnits=kg/m^3  Mass=15.195  MassUnits=g  CenterOfMass=[7.102 7.102 7.102]  CenterOfMassUnits=mm  MomentsOfInertia=[4.91955e-7 4.91955e-7 4.91955e-7]  MomentsOfInertiaUnits=kg*m^2  ProductsOfInertia=[2.9611e-8 2.9611e-8 2.9611e-8]  ProductsOfInertiaUnits=kg*m^2  GraphicType=FromGeometry  MarkerShape=Sphere  MarkerSize=10  GraphicVisPropType=SimpleVisualProperties  GraphicDiffuseColor=[0 0.7137 0.02353]  GraphicOpacity=1  GraphicSpecularColor=[0.5 0.5 0.5 1.0]  GraphicAmbientColor=[0.15 0.15 0.15 1.0]  GraphicEmissiveColor=[0.0 0.0 0.0 1.0]  GraphicShininess=75  DoExposeReferenceFrame=on  SerializedFrames=<Frames/>
  Cornerstone-b2 : sm_lib/Body Elements/File Solid  ExtGeomFileName=D:\Mechatronics\Non-Holonomical Cubli\GitHub Referance\balancing-cube-main\mechanical\models\cornerstone-b.step  UnitType=FromFile  ExtGeomFileUnits=m  StepReaderType=HEX  ExportConvexHullGeometry=on  InertiaType=Custom  BasedOnType=DensityFromFile  Density=1000  DensityUnits=kg/m^3  Mass=15.195  MassUnits=g  CenterOfMass=[7.102 7.102 7.102]  CenterOfMassUnits=mm  MomentsOfInertia=[4.91955e-7 4.91955e-7 4.91955e-7]  MomentsOfInertiaUnits=kg*m^2  ProductsOfInertia=[2.9611e-8 2.9611e-8 2.9611e-8]  ProductsOfInertiaUnits=kg*m^2  GraphicType=FromGeometry  MarkerShape=Sphere  MarkerSize=10  GraphicVisPropType=SimpleVisualProperties  GraphicDiffuseColor=[0 0.7137 0.02353]  GraphicOpacity=1  GraphicSpecularColor=[0.5 0.5 0.5 1.0]  GraphicAmbientColor=[0.15 0.15 0.15 1.0]  GraphicEmissiveColor=[0.0 0.0 0.0 1.0]  GraphicShininess=75  DoExposeReferenceFrame=on  SerializedFrames=<Frames/>
  Cornerstone-b3 : sm_lib/Body Elements/File Solid  ExtGeomFileName=D:\Mechatronics\Non-Holonomical Cubli\GitHub Referance\balancing-cube-main\mechanical\models\cornerstone-b.step  UnitType=FromFile  ExtGeomFileUnits=m  StepReaderType=HEX  ExportConvexHullGeometry=off  InertiaType=Custom  BasedOnType=DensityFromFile  Density=1000  DensityUnits=kg/m^3  Mass=15.195  MassUnits=g  CenterOfMass=[7.102 7.102 7.102]  CenterOfMassUnits=mm  MomentsOfInertia=[4.91955e-7 4.91955e-7 4.91955e-7]  MomentsOfInertiaUnits=kg*m^2  ProductsOfInertia=[2.9611e-8 2.9611e-8 2.9611e-8]  ProductsOfInertiaUnits=kg*m^2  GraphicType=FromGeometry  MarkerShape=Sphere  MarkerSize=10  GraphicVisPropType=SimpleVisualProperties  GraphicDiffuseColor=[0 0.7137 0.02353]  GraphicOpacity=1  GraphicSpecularColor=[0.5 0.5 0.5 1.0]  GraphicAmbientColor=[0.15 0.15 0.15 1.0]  GraphicEmissiveColor=[0.0 0.0 0.0 1.0]  GraphicShininess=75  DoExposeReferenceFrame=on  SerializedFrames=<Frames/>
  Cornerstone-b4 : sm_lib/Body Elements/File Solid  ExtGeomFileName=D:\Mechatronics\Non-Holonomical Cubli\GitHub Referance\balancing-cube-main\mechanical\models\cornerstone-b.step  UnitType=FromFile  ExtGeomFileUnits=m  StepReaderType=HEX  ExportConvexHullGeometry=off  InertiaType=Custom  BasedOnType=DensityFromFile  Density=1000  DensityUnits=kg/m^3  Mass=15.195  MassUnits=g  CenterOfMass=[7.102 7.102 7.102]  CenterOfMassUnits=mm  MomentsOfInertia=[4.91955e-7 4.91955e-7 4.91955e-7]  MomentsOfInertiaUnits=kg*m^2  ProductsOfInertia=[2.9611e-8 2.9611e-8 2.9611e-8]  ProductsOfInertiaUnits=kg*m^2  GraphicType=FromGeometry  MarkerShape=Sphere  MarkerSize=10  GraphicVisPropType=SimpleVisualProperties  GraphicDiffuseColor=[0 0.7137 0.02353]  GraphicOpacity=1  GraphicSpecularColor=[0.5 0.5 0.5 1.0]  GraphicAmbientColor=[0.15 0.15 0.15 1.0]  GraphicEmissiveColor=[0.0 0.0 0.0 1.0]  GraphicShininess=75  DoExposeReferenceFrame=on  SerializedFrames=<Frames/>
  Spatial Contact Force : sm_lib/Forces and Torques/Spatial Contact Force  SenseSeparationDistance=off  NormalForceType=SmoothSpringDamper  NormalStiffness=1e6  NormalStiffnessUnits=N/m  NormalDamping=1e3  NormalDampingUnits=N/(m/s)  NormalTransitionRegionWidth=1e-4  NormalTransitionRegionWidthUnits=m  FrictionType=SmoothStickSlip  CoefficientOfStaticFriction=0.5  CoefficientOfDynamicFriction=0.3  FrictionalCriticalVelocity=1e-3  FrictionalCriticalVelocityUnits=m/s  SenseContactSignal=off  SensePenetrationDepth=off  SenseNormalVelocity=off  SenseTangentialVelocity=off  SensingForceTorqueDirection=BaseOnFollower  SensingForceTorqueResolutionFrame=ContactFrame  SenseNormalForce=off  SenseNormalForceMagnitude=off  SenseNormalTorque=off  SenseFrictionalForce=off  SenseFrictionalForceMagnitude=off  SenseFrictionalTorque=off  SenseTotalForce=off  SenseTotalTorque=off  SenseContactBaseRotation=off  SenseContactBaseTranslation=off  SenseContactFollowerRotation=off  SenseContactFollowerTranslation=off  ZeroCrossDetectContactStartAndEnd=off
  Spatial Contact Force1 : sm_lib/Forces and Torques/Spatial Contact Force  SenseSeparationDistance=off  NormalForceType=SmoothSpringDamper  NormalStiffness=1e6  NormalStiffnessUnits=N/m  NormalDamping=1e3  NormalDampingUnits=N/(m/s)  NormalTransitionRegionWidth=1e-4  NormalTransitionRegionWidthUnits=m  FrictionType=SmoothStickSlip  CoefficientOfStaticFriction=0.5  CoefficientOfDynamicFriction=0.3  FrictionalCriticalVelocity=1e-3  FrictionalCriticalVelocityUnits=m/s  SenseContactSignal=off  SensePenetrationDepth=off  SenseNormalVelocity=off  SenseTangentialVelocity=off  SensingForceTorqueDirection=BaseOnFollower  SensingForceTorqueResolutionFrame=ContactFrame  SenseNormalForce=off  SenseNormalForceMagnitude=off  SenseNormalTorque=off  SenseFrictionalForce=off  SenseFrictionalForceMagnitude=off  SenseFrictionalTorque=off  SenseTotalForce=off  SenseTotalTorque=off  SenseContactBaseRotation=off  SenseContactBaseTranslation=off  SenseContactFollowerRotation=off  SenseContactFollowerTranslation=off  ZeroCrossDetectContactStartAndEnd=off
  Spatial Contact Force2 : sm_lib/Forces and Torques/Spatial Contact Force  SenseSeparationDistance=off  NormalForceType=SmoothSpringDamper  NormalStiffness=1e6  NormalStiffnessUnits=N/m  NormalDamping=1e3  NormalDampingUnits=N/(m/s)  NormalTransitionRegionWidth=1e-4  NormalTransitionRegionWidthUnits=m  FrictionType=SmoothStickSlip  CoefficientOfStaticFriction=0.5  CoefficientOfDynamicFriction=0.3  FrictionalCriticalVelocity=1e-3  FrictionalCriticalVelocityUnits=m/s  SenseContactSignal=off  SensePenetrationDepth=off  SenseNormalVelocity=off  SenseTangentialVelocity=off  SensingForceTorqueDirection=BaseOnFollower  SensingForceTorqueResolutionFrame=ContactFrame  SenseNormalForce=off  SenseNormalForceMagnitude=off  SenseNormalTorque=off  SenseFrictionalForce=off  SenseFrictionalForceMagnitude=off  SenseFrictionalTorque=off  SenseTotalForce=off  SenseTotalTorque=off  SenseContactBaseRotation=off  SenseContactBaseTranslation=off  SenseContactFollowerRotation=off  SenseContactFollowerTranslation=off  ZeroCrossDetectContactStartAndEnd=off
  World to cornerstone1 : sm_lib/Frames and Transforms/Rigid Transform  RotationMethod=StandardAxis  FollAlignAxisA=+X  BaseAlignAxisA=+Y  FollAlignAxisB=+Y  BaseAlignAxisB=+Z  RotationStandardAxis=+Z  RotationAngle=270  RotationAngleUnits=deg  RotationArbitraryAxis=[0 0 1]  RotationSequenceAxes=FollowerAxes  RotationSequence=ZXY  RotationSequenceAngles=[90 0 90]  RotationSequenceAnglesUnits=deg  RotationMatrix=[1 0 0;0 1 0;0 0 1]  Quaternion=[1 0 0 0]  TranslationMethod=Cartesian  TranslationCartesianOffset=[-75 75 0]  TranslationCartesianOffsetUnits=mm  TranslationStandardAxis=+Z  TranslationStandardOffset=0  TranslationStandardOffsetUnits=m  TranslationROffset=0  TranslationROffsetUnits=m  TranslationThetaOffset=0  TranslationThetaOffsetUnits=deg  TranslationZOffset=0  TranslationZOffsetUnits=m
  World to cornerstone2 : sm_lib/Frames and Transforms/Rigid Transform  RotationMethod=StandardAxis  FollAlignAxisA=+X  BaseAlignAxisA=+Y  FollAlignAxisB=+Y  BaseAlignAxisB=+Z  RotationStandardAxis=+Z  RotationAngle=0  RotationAngleUnits=deg  RotationArbitraryAxis=[0 0 1]  RotationSequenceAxes=FollowerAxes  RotationSequence=ZXY  RotationSequenceAngles=[90 0 90]  RotationSequenceAnglesUnits=deg  RotationMatrix=[1 0 0;0 1 0;0 0 1]  Quaternion=[1 0 0 0]  TranslationMethod=Cartesian  TranslationCartesianOffset=[-75 -75 0]  TranslationCartesianOffsetUnits=mm  TranslationStandardAxis=+Z  TranslationStandardOffset=0  TranslationStandardOffsetUnits=m  TranslationROffset=0  TranslationROffsetUnits=m  TranslationThetaOffset=0  TranslationThetaOffsetUnits=deg  TranslationZOffset=0  TranslationZOffsetUnits=m
  World to cornerstone3 : sm_lib/Frames and Transforms/Rigid Transform  RotationMethod=StandardAxis  FollAlignAxisA=+X  BaseAlignAxisA=+Y  FollAlignAxisB=+Y  BaseAlignAxisB=+Z  RotationStandardAxis=+Z  RotationAngle=90  RotationAngleUnits=deg  RotationArbitraryAxis=[0 0 1]  RotationSequenceAxes=FollowerAxes  RotationSequence=ZXY  RotationSequenceAngles=[90 0 90]  RotationSequenceAnglesUnits=deg  RotationMatrix=[1 0 0;0 1 0;0 0 1]  Quaternion=[1 0 0 0]  TranslationMethod=Cartesian  TranslationCartesianOffset=[75 -75 0]  TranslationCartesianOffsetUnits=mm  TranslationStandardAxis=+Z  TranslationStandardOffset=0  TranslationStandardOffsetUnits=m  TranslationROffset=0  TranslationROffsetUnits=m  TranslationThetaOffset=0  TranslationThetaOffsetUnits=deg  TranslationZOffset=0  TranslationZOffsetUnits=m
  World to cornerstone4 : sm_lib/Frames and Transforms/Rigid Transform  RotationMethod=StandardAxis  FollAlignAxisA=+X  BaseAlignAxisA=+Y  FollAlignAxisB=+Y  BaseAlignAxisB=+Z  RotationStandardAxis=+Y  RotationAngle=180  RotationAngleUnits=deg  RotationArbitraryAxis=[0 0 1]  RotationSequenceAxes=FollowerAxes  RotationSequence=ZXY  RotationSequenceAngles=[90 0 90]  RotationSequenceAnglesUnits=deg  RotationMatrix=[1 0 0;0 1 0;0 0 1]  Quaternion=[1 0 0 0]  TranslationMethod=Cartesian  TranslationCartesianOffset=[75 -75 150]  TranslationCartesianOffsetUnits=mm  TranslationStandardAxis=+Z  TranslationStandardOffset=0  TranslationStandardOffsetUnits=m  TranslationROffset=0  TranslationROffsetUnits=m  TranslationThetaOffset=0  TranslationThetaOffsetUnits=deg  TranslationZOffset=0  TranslationZOffsetUnits=m
  World to cornerstone5 : sm_lib/Frames and Transforms/Rigid Transform  RotationMethod=RotationSequence  FollAlignAxisA=+X  BaseAlignAxisA=+Y  FollAlignAxisB=+Y  BaseAlignAxisB=+Z  RotationStandardAxis=+Z  RotationAngle=270  RotationAngleUnits=deg  RotationArbitraryAxis=[0 0 1]  RotationSequenceAxes=FollowerAxes  RotationSequence=YXZ  RotationSequenceAngles=[90 180 0]  RotationSequenceAnglesUnits=deg  RotationMatrix=[1 0 0;0 1 0;0 0 1]  Quaternion=[1 0 0 0]  TranslationMethod=Cartesian  TranslationCartesianOffset=[75 75 150]  TranslationCartesianOffsetUnits=mm  TranslationStandardAxis=+Z  TranslationStandardOffset=0  TranslationStandardOffsetUnits=m  TranslationROffset=0  TranslationROffsetUnits=m  TranslationThetaOffset=0  TranslationThetaOffsetUnits=deg  TranslationZOffset=0  TranslationZOffsetUnits=m
  World to cornerstone6 : sm_lib/Frames and Transforms/Rigid Transform  RotationMethod=StandardAxis  FollAlignAxisA=+X  BaseAlignAxisA=+Y  FollAlignAxisB=+Y  BaseAlignAxisB=+Z  RotationStandardAxis=+X  RotationAngle=180  RotationAngleUnits=deg  RotationArbitraryAxis=[0 0 1]  RotationSequenceAxes=FollowerAxes  RotationSequence=ZXY  RotationSequenceAngles=[90 0 90]  RotationSequenceAnglesUnits=deg  RotationMatrix=[1 0 0;0 1 0;0 0 1]  Quaternion=[1 0 0 0]  TranslationMethod=Cartesian  TranslationCartesianOffset=[-75 75 150]  TranslationCartesianOffsetUnits=mm  TranslationStandardAxis=+Z  TranslationStandardOffset=0  TranslationStandardOffsetUnits=m  TranslationROffset=0  TranslationROffsetUnits=m  TranslationThetaOffset=0  TranslationThetaOffsetUnits=deg  TranslationZOffset=0  TranslationZOffsetUnits=m
  World to cornerstone7 : sm_lib/Frames and Transforms/Rigid Transform  RotationMethod=StandardAxis  FollAlignAxisA=+X  BaseAlignAxisA=+Y  FollAlignAxisB=+Y  BaseAlignAxisB=+Z  RotationStandardAxis=+Y  RotationAngle=90  RotationAngleUnits=deg  RotationArbitraryAxis=[0 0 1]  RotationSequenceAxes=FollowerAxes  RotationSequence=ZXY  RotationSequenceAngles=[90 0 90]  RotationSequenceAnglesUnits=deg  RotationMatrix=[1 0 0;0 1 0;0 0 1]  Quaternion=[1 0 0 0]  TranslationMethod=Cartesian  TranslationCartesianOffset=[-75 -75 150]  TranslationCartesianOffsetUnits=mm  TranslationStandardAxis=+Z  TranslationStandardOffset=0  TranslationStandardOffsetUnits=m  TranslationROffset=0  TranslationROffsetUnits=m  TranslationThetaOffset=0  TranslationThetaOffsetUnits=deg  TranslationZOffset=0  TranslationZOffsetUnits=m
  W to C : PMIOPort  Side=Left
  Spatial Contact : PMIOPort  Port=2  Side=Right
  connections:
  Cornerstone-a1/RConn1 -- World to cornerstone1/RConn1
  World to cornerstone7/LConn1 -- W to C/RConn1 -- World to cornerstone4/LConn1 -- World to cornerstone3/LConn1 -- World to cornerstone1/LConn1 -- World to cornerstone2/LConn1 -- World to cornerstone5/LConn1 -- World to cornerstone6/LConn1
  Cornerstone-a2/RConn1 -- World to cornerstone3/RConn1
  Cornerstone-b4/RConn1 -- World to cornerstone6/RConn1
  Cornerstone-b2/RConn1 -- World to cornerstone2/RConn1
  Cornerstone-b3/RConn1 -- World to cornerstone4/RConn1
  Cornerstone-a4/RConn1 -- World to cornerstone7/RConn1
  Cornerstone-a3/RConn1 -- World to cornerstone5/RConn1
  Spatial Contact/RConn1 -- Spatial Contact Force1/LConn1 -- Spatial Contact Force2/LConn1 -- Spatial Contact Force/LConn1
  Spatial Contact Force/RConn1 -- Cornerstone-a2/LConn1
  Cornerstone-b2/LConn1 -- Spatial Contact Force1/RConn1
  Spatial Contact Force2/RConn1 -- Cornerstone-a1/LConn1

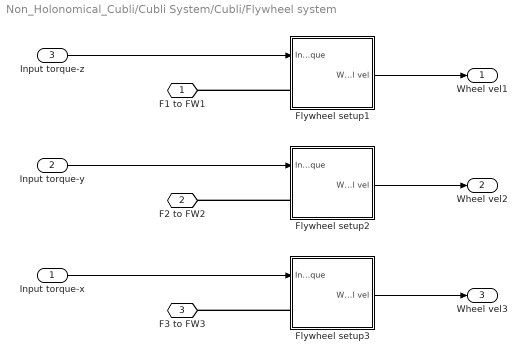
== system Non_Holonomical_Cubli/Cubli System/Cubli/Flywheel system ==
  Input torque-x : Inport
  Input torque-y : Inport  Port=2
  Input torque-z : Inport  Port=3
  Flywheel setup1 : Subsystem
  Flywheel setup2 : Subsystem
  Flywheel setup3 : Subsystem
  F1 to FW1 : PMIOPort  Side=Left
  F2 to FW2 : PMIOPort  Port=2  Side=Left
  F3 to FW3 : PMIOPort  Port=3  Side=Left
  Wheel vel1 : Outport
  Wheel vel2 : Outport  Port=2
  Wheel vel3 : Outport  Port=3
  wires:
  Input torque-z/1 -> Flywheel setup1/1(Input torque)
  Flywheel setup1/1(Wheel vel) -> Wheel vel1/1
  Input torque-y/1 -> Flywheel setup2/1(Input torque)
  Flywheel setup2/1(Wheel vel) -> Wheel vel2/1
  Input torque-x/1 -> Flywheel setup3/1(Input torque)
  Flywheel setup3/1(Wheel vel) -> Wheel vel3/1
  connections:
  Flywheel setup2/LConn1 -- F2 to FW2/RConn1
  Flywheel setup1/LConn1 -- F1 to FW1/RConn1
  Flywheel setup3/LConn1 -- F3 to FW3/RConn1

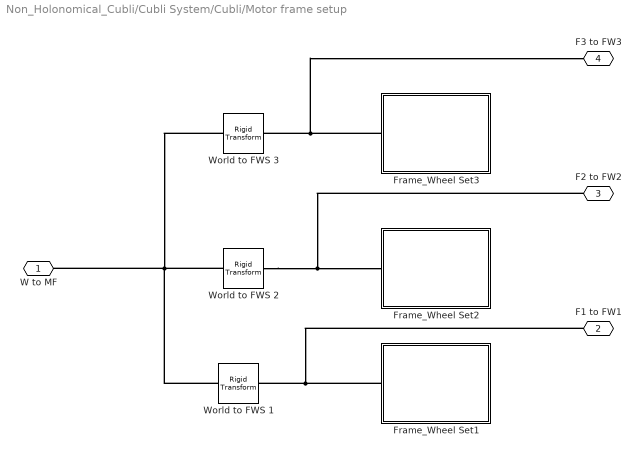
== system Non_Holonomical_Cubli/Cubli System/Cubli/Motor frame setup ==
  Frame_Wheel Set1 : Subsystem
  Frame_Wheel Set2 : Subsystem
  Frame_Wheel Set3 : Subsystem
  World to FWS 1 : sm_lib/Frames and Transforms/Rigid Transform  RotationMethod=None  FollAlignAxisA=+X  BaseAlignAxisA=+Y  FollAlignAxisB=+Y  BaseAlignAxisB=+Z  RotationStandardAxis=+Z  RotationAngle=0  RotationAngleUnits=deg  RotationArbitraryAxis=[0 0 1]  RotationSequenceAxes=FollowerAxes  RotationSequence=XYX  RotationSequenceAngles=[0 0 0]  RotationSequenceAnglesUnits=deg  RotationMatrix=[1 0 0;0 1 0;0 0 1]  Quaternion=[1 0 0 0]  TranslationMethod=Cartesian  TranslationCartesianOffset=[75 75 0]  TranslationCartesianOffsetUnits=mm  TranslationStandardAxis=+Z  TranslationStandardOffset=0  TranslationStandardOffsetUnits=m  TranslationROffset=0  TranslationROffsetUnits=m  TranslationThetaOffset=0  TranslationThetaOffsetUnits=deg  TranslationZOffset=0  TranslationZOffsetUnits=m
  World to FWS 2 : sm_lib/Frames and Transforms/Rigid Transform  RotationMethod=RotationSequence  FollAlignAxisA=+X  BaseAlignAxisA=+Y  FollAlignAxisB=+Y  BaseAlignAxisB=+Z  RotationStandardAxis=+Y  RotationAngle=90  RotationAngleUnits=deg  RotationArbitraryAxis=[0 0 1]  RotationSequenceAxes=FollowerAxes  RotationSequence=ZXY  RotationSequenceAngles=[-90 0 -90]  RotationSequenceAnglesUnits=deg  RotationMatrix=[1 0 0;0 1 0;0 0 1]  Quaternion=[1 0 0 0]  TranslationMethod=Cartesian  TranslationCartesianOffset=[75 0 75]  TranslationCartesianOffsetUnits=mm  TranslationStandardAxis=+Z  TranslationStandardOffset=0  TranslationStandardOffsetUnits=m  TranslationROffset=0  TranslationROffsetUnits=m  TranslationThetaOffset=0  TranslationThetaOffsetUnits=deg  TranslationZOffset=0  TranslationZOffsetUnits=m
  World to FWS 3 : sm_lib/Frames and Transforms/Rigid Transform  RotationMethod=RotationSequence  FollAlignAxisA=+X  BaseAlignAxisA=+Y  FollAlignAxisB=+Y  BaseAlignAxisB=+Z  RotationStandardAxis=+Y  RotationAngle=90  RotationAngleUnits=deg  RotationArbitraryAxis=[0 0 1]  RotationSequenceAxes=FollowerAxes  RotationSequence=ZXY  RotationSequenceAngles=[90 90 0]  RotationSequenceAnglesUnits=deg  RotationMatrix=[1 0 0;0 1 0;0 0 1]  Quaternion=[1 0 0 0]  TranslationMethod=Cartesian  TranslationCartesianOffset=[0 75 75]  TranslationCartesianOffsetUnits=mm  TranslationStandardAxis=+Z  TranslationStandardOffset=0  TranslationStandardOffsetUnits=m  TranslationROffset=0  TranslationROffsetUnits=m  TranslationThetaOffset=0  TranslationThetaOffsetUnits=deg  TranslationZOffset=0  TranslationZOffsetUnits=m
  W to MF : PMIOPort  Side=Left
  F1 to FW1 : PMIOPort  Port=2  Side=Right
  F2 to FW2 : PMIOPort  Port=3  Side=Right
  F3 to FW3 : PMIOPort  Port=4  Side=Right
  connections:
  Frame_Wheel Set3/LConn1 -- F3 to FW3/RConn1 -- World to FWS 3/RConn1
  World to FWS 2/LConn1 -- World to FWS 1/LConn1 -- W to MF/RConn1 -- World to FWS 3/LConn1
  World to FWS 2/RConn1 -- F2 to FW2/RConn1 -- Frame_Wheel Set2/LConn1
  Frame_Wheel Set1/LConn1 -- F1 to FW1/RConn1 -- World to FWS 1/RConn1

== system Non_Holonomical_Cubli/Cubli System/Cubli/Non-Motor frame setup ==
  Nonmotor frame 1 : Subsystem
  Nonmotor frame 2 : Subsystem
  Nonmotor frame 3 : Subsystem
  W to NMF : PMIOPort  Side=Left
  connections:
  Nonmotor frame 3/LConn1 -- Nonmotor frame 1/LConn1 -- W to NMF/RConn1 -- Nonmotor frame 2/LConn1

== system Non_Holonomical_Cubli/Master Controller/Edge_Balance_Torque/jump_switch ==
  theta_angle : Inport
  1 degree : simulink/Logic and Bit Operations/Compare To Constant  relop=<=  const=0.02  OutDataTypeStr=boolean
  Data Type Conversion : DataTypeConversion  SaturateOnIntegerOverflow=off  RndMeth=Floor
  Demux : Demux  Outputs=3
  Integrator : Integrator
  S-R Flip-Flop1 : simulink_extras/Flip Flops/S-R Flip-Flop  initial_condition=0
  timmer : Outport
  wires:
  1 degree/1 -> S-R Flip-Flop1/1
  theta_angle/1 -> Demux/1
  S-R Flip-Flop1/1 -> Data Type Conversion/1
  Integrator/1 -> timmer/1
  Demux/2 -> 1 degree/1
  Data Type Conversion/1 -> Integrator/1
